simulink model "cyl_sim"  (Simulink 8.3)
settings: Solver=ode45  StartTime=0.0  StopTime=30  RelTol=1e-6  AbsTol=1e-6
values from neighbouring files (symbols this model uses):
  B = Orig_B+(percent_change_in_B/100*Orig_B)    (= 51.9540885087)    [init.m]
  cb = cb*scale    [final_plot_cyl.m]    (also in init.m = [0 0  -0.1])
  cg = cg*scale    [final_plot_cyl.m]    (also in init.m = [0 0  0.1])
  height = 0.3    [init.m]
  m = W/9.8    (= 5.30143760293)    [init.m]
  q0 = [10 10 10 10*deg_to_rad 0*deg_to_rad 0*deg_to_rad 0 0 0 0*deg_to_rad 0*deg_to_rad 0*deg_to_rad]    [init.m]
  rad = dia/2    (= 0.075)    [init.m]
  rho_water = 1000    [init.m]
  W = Orig_B    (= 51.9540885087)    [init.m]
settings Model: Creator=Owner  LastModifiedBy=Dr. Asokan
settings OptimizationCC: ExpressionDepthLimit=2147483647
settings DebuggingCC: FcnCallInpInsideContextMsg=EnableAllAsWarning
settings RTWCC: RTWCompilerOptimization=On
settings GRTTargetCC: CombineOutputUpdateFcns=on  GRTInterface=off

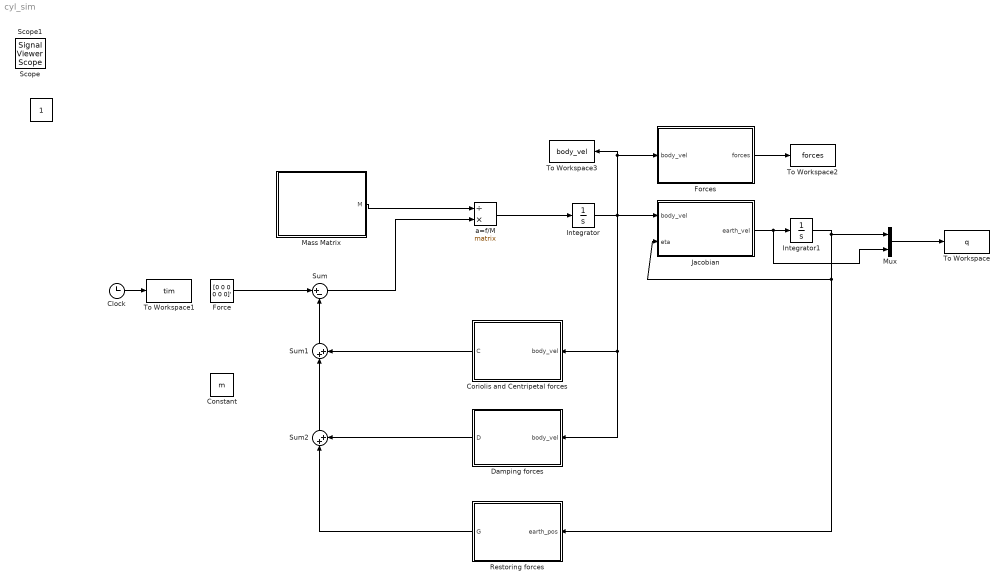
== system cyl_sim ==
  Clock : Clock
  Constant : Constant  Value=m
  Coriolis and Centripetal forces : MATLAB Function  TreatAsAtomicUnit=on
  Damping forces : MATLAB Function  TreatAsAtomicUnit=on
  Force : Constant  Value=[0 0 0 0 0 0]'
  Forces : MATLAB Function  TreatAsAtomicUnit=on
  Integrator : Integrator  InitialCondition=q0(7:12)'  ContinuousStateAttributes='velocities'
  Integrator1 : Integrator  InitialCondition=q0(1:6)'  ZeroCross=off
  Jacobian : MATLAB Function  TreatAsAtomicUnit=on
  Mass Matrix : MATLAB Function  TreatAsAtomicUnit=on
  Mux : Mux  Inputs=2
  Restoring forces : MATLAB Function  TreatAsAtomicUnit=on
  Sum : Sum  Inputs=|+-
  Sum1 : Sum  Inputs=|++
  Sum2 : Sum  Inputs=|++
  To Workspace : ToWorkspace  VariableName=q  SampleTime=-1
  To Workspace1 : ToWorkspace  VariableName=tim  SampleTime=-1
  To Workspace2 : ToWorkspace  VariableName=forces  SampleTime=-1
  To Workspace3 : ToWorkspace  VariableName=body_vel  SampleTime=-1
  a=f/M : Product  Inputs=/*  Multiplication=Matrix(*)
  "      " : Constant  IOType=siggen
  Scope : SignalViewerScope  IOType=viewer  RefreshTime=0.035000
      settings: ShowLegends=on
  Scope1 : SignalViewerScope  IOType=viewer  RefreshTime=0.035000
      settings: ShowLegends=on
  wires:
  a=f/M/1 -> Integrator/1
  Integrator/1 -> To Workspace3/1, Forces/1(body_vel), Jacobian/1(body_vel), Damping forces/1(body_vel), Coriolis and Centripetal forces/1(body_vel)
  Mass Matrix/1(M) -> a=f/M/1
  Jacobian/1(earth_vel) -> Mux/2, Integrator1/1
  Force/1 -> Sum/1
  Sum/1 -> a=f/M/2
  Coriolis and Centripetal forces/1(C) -> Sum1/2
  Sum1/1 -> Sum/2
  Damping forces/1(D) -> Sum2/2
  Sum2/1 -> Sum1/1
  Restoring forces/1(G) -> Sum2/1
  Integrator1/1 -> Mux/1, Restoring forces/1(earth_pos), Jacobian/2(eta)
  Mux/1 -> To Workspace/1
  Clock/1 -> To Workspace1/1
  Forces/1(forces) -> To Workspace2/1

== matlab function Coriolis and Centripetal forces ==
  data: C output double; body_vel input double; m parameter double; cg parameter double; rho_water parameter double; rad parameter double; height parameter double
function C = Coriolis_Centripetal(body_vel, m, cg, rho_water, rad, height)


xg=cg(1);
yg=cg(2);
zg=cg(3);

Ix = m*(3*(rad^2)+(height^2))/12;
Iy = m*(3*(rad^2)+(height^2))/12;
Iz = (m*rad^2)/2;
Ixy = 0;Ixz = 0;Iyx = 0;Iyz = 0;Izx = 0;Izy = 0;

u=body_vel(1);
v=body_vel(2);
w=body_vel(3);
p=body_vel(4);
q=body_vel(5);
r=body_vel(6);

xudot = -pi*rho_water*(rad^2)*height;
yvdot = -pi*rho_water*(rad^2)*height;
zwdot = -0.1*m;
kpdot = -(pi/12)*rho_water*(rad^2)*(height^3);
mqdot = -(pi/12)*rho_water*(rad^2)*(height^3);
nrdot =  0;

C_rb= [ 0              0              0              m*(yg*q+zg*r)    -m*(xg*q-w)       -m*(xg*r+v);
        0              0              0             -m*(yg*p+w)        m*(zg*r+xg*p)    -m*(yg*r-u);
        0              0              0             -m*(zg*p-v)       -m*(zg*q+u)        m*(xg*p+yg*q);
       -m*(yg*q+zg*r)  m*(yg*p+w)     m*(zg*p-v)     0                -Iyz*q-Ixz*p+Iz*r  Iyz*r+Ixy*p-Iy*q;
        m*(xg*q-w)    -m*(zg*r+xg*p)  m*(zg*q+u)     Iyz*q+Ixz*p-Iz*r  0                -Ixz*r-Ixy*q+Ix*p;
        m*(xg*r+v)     m*(yg*r-u)    -m*(xg*p+yg*q) -Iyz*r-Ixy*p+Iy*q  Ixz*r+Ixy*q-Ix*p  0];
    
    
C_a = [ 0        0        0        0       -zwdot*w  yvdot*v;
        0        0        0        zwdot*w  0       -xudot*u;
        0        0        0       -yvdot*v  xudot*u  0;
        0       -zwdot*w  yvdot*v  0       -nrdot*r  mqdot*q;
        zwdot*w  0       -xudot*u  nrdot*r  0       -kpdot*p;
       -yvdot*v  xudot*u  0       -mqdot*q  kpdot*p  0];

C_mat = C_rb + C_a;

C = C_mat * body_vel;

end

== matlab function Mass Matrix ==
  data: M output double; m parameter double; cg parameter double; rho_water parameter double; rad parameter double; height parameter double
function M = Mass_matrix(m, cg, rho_water, rad, height)

xg=cg(1);
yg=cg(2);
zg=cg(3);

Ix = m*(3*(rad^2)+(height^2))/12;
Iy = m*(3*(rad^2)+(height^2))/12;
Iz = (m*rad^2)/2;
Ixy = 0;Ixz = 0;Iyx = 0;Iyz = 0;Izx = 0;Izy = 0;

M_rb=[ m     0     0     0     m*zg -m*yg;
       0     m     0    -m*zg  0     m*xg;
       0     0     m     m*yg -m*xg  0;
       0    -m*zg  m*yg  Ix   -Ixy  -Ixz;
       m*zg  0    -m*xg -Iyx   Iy   -Iyz;
      -m*yg  m*xg  0    -Izx  -Izy   Iz];
  
xudot = -pi*rho_water*(rad^2)*height;
yvdot = -pi*rho_water*(rad^2)*height;
zwdot = -0.1*m;
kpdot = -pi/12*rho_water*(rad^2)*height^3;
mqdot = -pi/12*rho_water*(rad^2)*height^3;
nrdot =  0;

M_a = -[xudot 0     0     0     0     0;
        0     yvdot 0     0     0     0;
        0     0     zwdot 0     0     0;
        0     0     0     kpdot 0     0;
        0     0     0     0     mqdot 0;
        0     0     0     0     0     nrdot];
    
M = M_rb + M_a;

end

== matlab function Restoring forces ==
  data: G output double; earth_pos input double; cg parameter double; cb parameter double; W parameter double; B parameter double
function G = Restoring_Forces(earth_pos, cg, cb, W, B)

phi   = earth_pos(4);
theta = earth_pos(5);

xg=cg(1);
yg=cg(2);
zg=cg(3);

xb=cb(1);
yb=cb(2);
zb=cb(3);


G = [  (W-B)*sin(theta);
      -(W-B)*cos(theta)*sin(phi);
      -(W-B)*cos(theta)*cos(phi);
      -(yg*W-yb*B)*cos(theta)*cos(phi)+(zg*W-zb*B)*cos(theta)*sin(phi);
       (zg*W-zb*B)*sin(theta)+(xg*W-xb*B)*cos(theta)*cos(phi);
      -(xg*W-xb*B)*cos(theta)*sin(phi)-(yg*W-yb*B)*sin(theta)];

end

== matlab function Jacobian ==
  data: earth_vel output double; body_vel input double; eta input double
function earth_vel = Jacobian(body_vel,eta)

phi=eta(4);
theta=eta(5);
si=eta(6);

c_p=cos(phi);
c_t=cos(theta);
c_s=cos(si);
s_p=sin(phi);
s_t=sin(theta);
s_s=sin(si);
t_t=tan(theta);


J1=[c_s*c_t    -s_s*c_p+s_p*s_t*c_s     s_s*s_p+s_t*c_s*c_p;
    s_s*c_t     c_s*c_p+s_p*s_t*s_s    -c_s*s_p+s_t*s_s*c_p;
     -s_t            s_p*c_t                 c_p*c_t       ];
       
J2=[1      s_p*t_t     c_p*t_t;
    0        c_p        -s_p;
    0      s_p/c_t     c_p/c_t ];


J=[J1 zeros(3,3); zeros(3,3) J2];

earth_vel = J * body_vel;

end

== matlab function Damping forces ==
  data: D output double; body_vel input double
function D = Damping(body_vel)

u=body_vel(1);
v=body_vel(2);
w=body_vel(3);

U=sqrt(u^2+v^2+w^2);

% D_mat = U*[5+27*abs(u) 0           0           0   0   0;
%        0           5+27*abs(v) 0           0   0   0;
%        0           0           2+27*abs(w) 0   0   0;
%        0           0           0           200 0   0;
%        0           0           0           0   200 0;
%        0           0           0           0   0   100];

D_mat = U*[1+7*abs(u)  0           0           0   0   0;
           0           1+7*abs(v)  0           0   0   0;
           0           0           1+5*abs(w)  0   0   0;
           0           0           0           20  0   0;
           0           0           0           0   20  0;
           0           0           0           0   0   10];
%        
D = D_mat * body_vel;

end

== matlab function Forces ==
  data: forces output double; body_vel input double; m parameter double; cg parameter double; rho_water parameter double; rad parameter double; height parameter double
function forces = forces_drag(body_vel, m, cg, rho_water, rad, height)

u=body_vel(1);
v=body_vel(2);
w=body_vel(3);

x_force = 0.5*rho_water*2*rad*height*1.2*u*abs(u);
y_force = 0.5*rho_water*2*rad*height*1.2*v*abs(v);
z_force = 0.5*rho_water*pi*(rad^2)*1.2*w*abs(w);

forces = [x_force y_force z_force]';

end
